simulink model "EngineAirMassFlow"  (R2025b)
settings: Solver=VariableStepAuto  StartTime=0.0  StopTime=10.0  RelTol=1e-3
values from neighbouring files (symbols this model uses):
  R = 287    [Throttle_Parameter_Identification.m]
undefined symbols (not defined in the file or in its folder): gamma_0, gamma_1, kappa, lambda, sigma_0, Vc, Vd
settings Model: Creator=khanh  LastModifiedBy=khanh

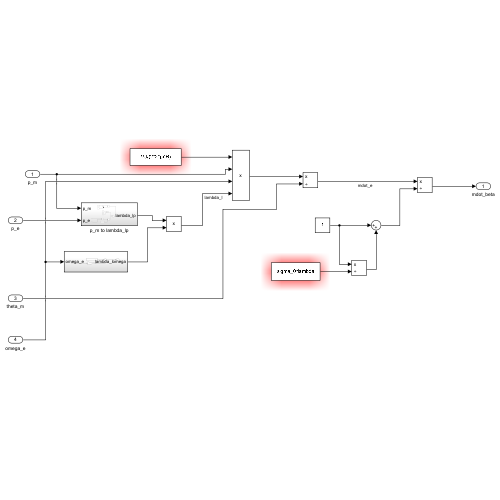
[thumbnail: Simulink's stored preview of the top-level diagram]
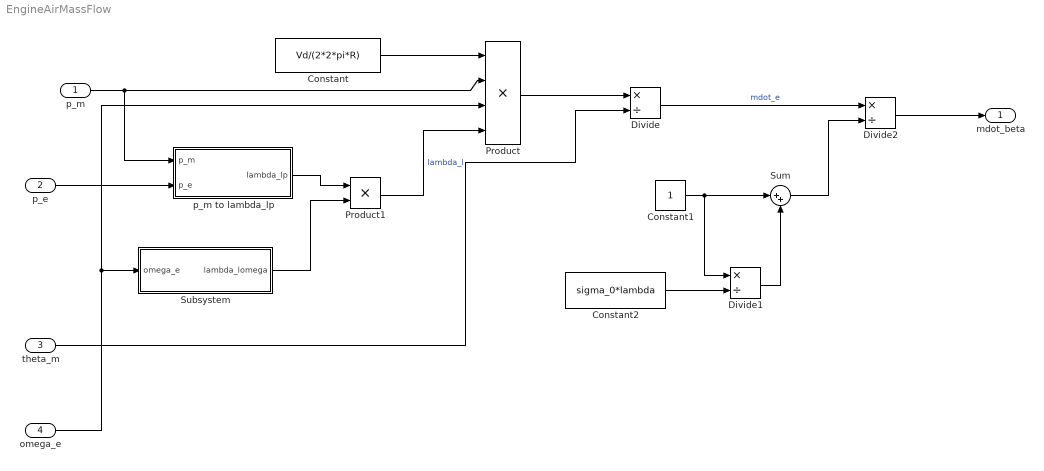
== system EngineAirMassFlow ==
  p_m : Inport
  p_e : Inport  Port=2
  theta_m : Inport  Port=3
  omega_e : Inport  Port=4
  Constant : Constant  Value=Vd/(2*2*pi*R)
  Constant1 : Constant
  Constant2 : Constant  Value=sigma_0*lambda
  Divide : Product  Inputs=*/
  Divide1 : Product  Inputs=*/
  Divide2 : Product  Inputs=*/
  Product : Product  Inputs=4
  Product1 : Product
  Subsystem : Subsystem
  Sum : Sum  Inputs=|++
  p_m to lambda_lp : Subsystem
  mdot_beta : Outport
  wires:
  p_m/1 -> p_m to lambda_lp/1(p_m), Product/2
  Constant/1 -> Product/1
  omega_e/1 -> Product/3, Subsystem/1(omega_e)
  Product1/1 -> Product/4  "lambda_l"
  Product/1 -> Divide/1
  theta_m/1 -> Divide/2
  Divide/1 -> Divide2/1  "mdot_e"
  Constant1/1 -> Divide1/1, Sum/1
  Constant2/1 -> Divide1/2
  Divide1/1 -> Sum/2
  Sum/1 -> Divide2/2
  Divide2/1 -> mdot_beta/1
  p_e/1 -> p_m to lambda_lp/2(p_e)
  Subsystem/1(lambda_lomega) -> Product1/2
  p_m to lambda_lp/1(lambda_lp) -> Product1/1

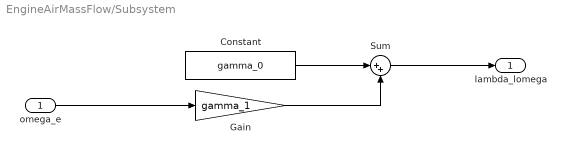
== system EngineAirMassFlow/Subsystem ==
  omega_e : Inport
  Constant : Constant  Value=gamma_0
  Gain : Gain  Gain=gamma_1
  Sum : Sum  Inputs=|++
  lambda_lomega : Outport
  wires:
  Constant/1 -> Sum/1
  omega_e/1 -> Gain/1
  Gain/1 -> Sum/2
  Sum/1 -> lambda_lomega/1

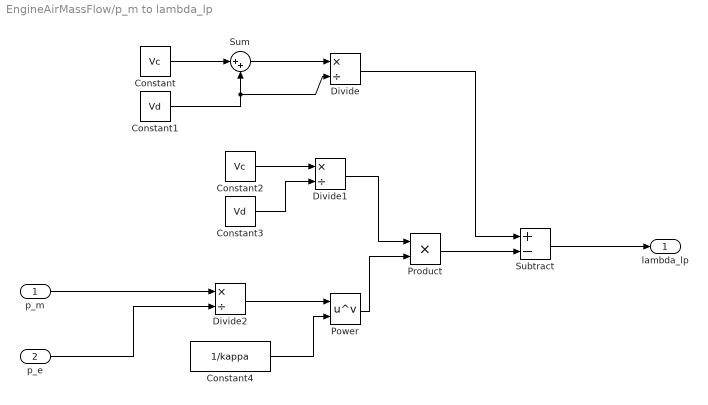
== system EngineAirMassFlow/p_m to lambda_lp ==
  p_m : Inport
  p_e : Inport  Port=2
  Constant : Constant  Value=Vc
  Constant1 : Constant  Value=Vd
  Constant2 : Constant  Value=Vc
  Constant3 : Constant  Value=Vd
  Constant4 : Constant  Value=1/kappa
  Divide : Product  Inputs=*/
  Divide1 : Product  Inputs=*/
  Divide2 : Product  Inputs=*/
  Power : Math  Operator=pow
  Product : Product
  Subtract : Sum  Inputs=+-
  Sum : Sum  Inputs=|++
  lambda_lp : Outport
  wires:
  Constant/1 -> Sum/1
  Constant1/1 -> Sum/2, Divide/2
  Sum/1 -> Divide/1
  Constant2/1 -> Divide1/1
  Constant3/1 -> Divide1/2
  p_m/1 -> Divide2/1
  p_e/1 -> Divide2/2
  Divide2/1 -> Power/1
  Constant4/1 -> Power/2
  Divide1/1 -> Product/1
  Power/1 -> Product/2
  Divide/1 -> Subtract/1
  Product/1 -> Subtract/2
  Subtract/1 -> lambda_lp/1
